simulink model "Planta_Controle_em_Espaco_de_Estados"  (Simulink 8.7)
settings: Solver=VariableStepAuto  StartTime=0.0  StopTime=40  RelTol=1e-3
settings Model: Creator=Tiago  LastModifiedBy=Tiago  NumberOfSteps=10
settings DataIOCC: LimitDataPoints=off  SaveFormat=Dataset
settings DebuggingCC: UnderspecifiedInitializationDetection=Simplified  MergeDetectMultiDrivingBlocksExec=error
settings HardwareCC: ProdBitPerPointer=64  ProdLargestAtomicFloat=Float  ProdIntDivRoundTo=Zero  ProdEndianess=LittleEndian  ProdWordSize=64  ProdHWDeviceType=Intel->x86-64 (Windows64)
settings ModelReferenceCC: PropagateSignalLabelsOutOfModel=on
settings ConfigComp: CovModelRefEnable=off

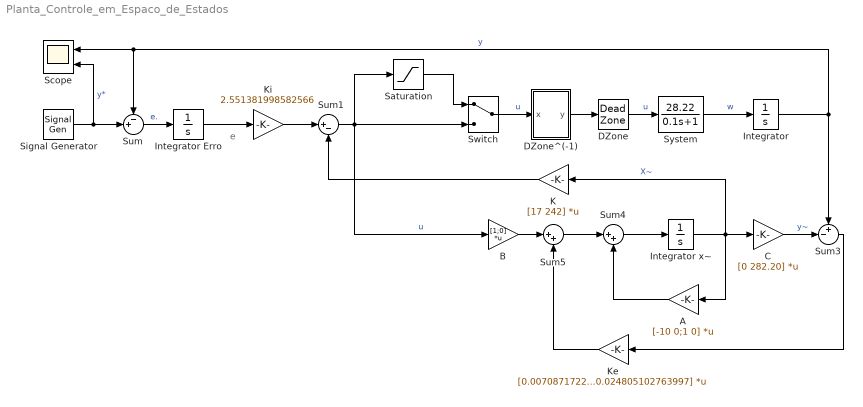
== system Planta_Controle_em_Espaco_de_Estados ==
  note: e
  A : Gain  Gain=[-10 0;1 0]  Multiplication=Matrix(K*u)
  B : Gain  Gain=[1;0]  Multiplication=Matrix(K*u)
  C : Gain  Gain=[0 282.20]  Multiplication=Matrix(K*u)
  DZone : DeadZone  LowerValue=-0.5296  UpperValue=0.5635  SaturateOnIntegerOverflow=on
  DZone^(-1) : MATLAB Function  TreatAsAtomicUnit=on
  Integrator : Integrator
  Integrator Erro : Integrator
  Integrator x~ : Integrator
  K : Gain  Gain=[17 242]  Multiplication=Matrix(K*u)
  Ke : Gain  Gain=[0.007087172218285;0.024805102763997]  Multiplication=Matrix(K*u)
  Ki : Gain  Gain=2.551381998582566
  Saturation : Saturate  UpperLimit=10  LowerLimit=-10
  Scope : Scope  NumInputPorts=2
  Signal Generator : SignalGenerator  WaveForm=square  Amplitude=45  Frequency=0.5  Units=rad/sec
  Sum : Sum  Inputs=-+|
  Sum1 : Sum  Inputs=|+-
  Sum3 : Sum  Inputs=+-|
  Sum4 : Sum  Inputs=|++
  Sum5 : Sum  Inputs=|++
  Switch : ManualSwitch
  System : TransferFcn  Numerator=[28.22]  Denominator=[0.1 1]
  wires:
  Signal Generator/1 -> Scope/2, Sum/2  "y*"
  Sum1/1 -> B/1, Switch/2, Saturation/1  "u"
  K/1 -> Sum1/2
  Integrator Erro/1 -> Ki/1
  Ki/1 -> Sum1/1
  Integrator/1 -> Sum3/1, Scope/1, Sum/1  "y"
  C/1 -> Sum3/2  "y~"
  Integrator x~/1 -> K/1, A/1, C/1  "X~"
  Sum4/1 -> Integrator x~/1
  A/1 -> Sum4/2
  B/1 -> Sum5/1
  Sum5/1 -> Sum4/1
  Sum3/1 -> Ke/1
  Ke/1 -> Sum5/2
  Sum/1 -> Integrator Erro/1  "e."
  System/1 -> Integrator/1  "w"
  Switch/1 -> DZone^(-1)/1(x)  "u"
  Saturation/1 -> Switch/1
  DZone^(-1)/1(y) -> DZone/1
  DZone/1 -> System/1  "u"

== matlab function DZone^(-1) ==
  data: x input double; y output double
function y = fcn(x)
    if(x > 0)
        x = x + 0.5635;
    elseif (x < 0) 
        x = x - 0.5296;
    else 
        x = 0;
    end
y = x;
